simulink model "sf_ladder_logic_scheduler"  (Simulink 7.6)
settings: Solver=FixedStepDiscrete  StartTime=0.0  StopTime=10  RelTol=1e-3
model workspace (MAT data in the model file):
  deltat : Simulink.Parameter (value not decoded)
settings Model: Creator=The MathWorks Inc.
settings SolverCC: InsertRTBMode=Auto
settings OptimizationCC: InitFltsAndDblsToZero=on
settings DebuggingCC: SaveWithParameterizedLinksMsg=none  SignalResolutionControl=TryResolveAllWithWarning  InheritedTsInSrcMsg=none  MultiTaskDSMMsg=warning  MultiTaskCondExecSysMsg=none  StrictBusMsg=None
settings SFSimCC: SFSimEcho=off  SimParseCustomCode=off
settings RTWCC: IncludeERTFirstTime=on
settings GRTTargetCC: TargetFcnLib=ansi_tfl_tmw.mat

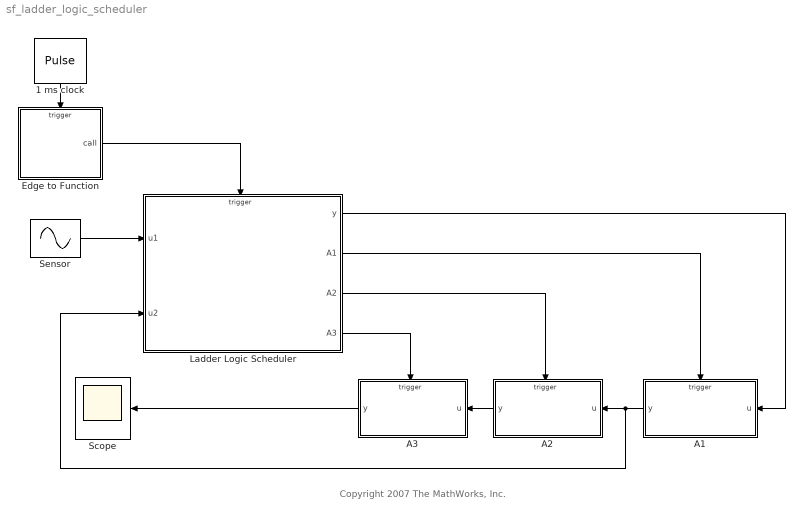
== system sf_ladder_logic_scheduler ==
  note: Copyright 2007 The MathWorks, Inc.
  1 ms clock : DiscretePulseGenerator  PulseType=Time based  Period=0.001  PulseWidth=10
  A1 : Subsystem  TreatAsAtomicUnit=on
  A2 : Subsystem  TreatAsAtomicUnit=on
  A3 : Subsystem  TreatAsAtomicUnit=on
  "Edge to Function " : Stateflow chart  TreatAsAtomicUnit=on
  Ladder Logic Scheduler : Stateflow chart  TreatAsAtomicUnit=on
  Scope : Scope
      settings: TimeRange=0.5  YMin=0  YMax=2
  Sensor : Sin  Frequency=40  Phase=-pi/8
  wires:
  Ladder Logic Scheduler/1(y) -> A1/1(u)
  Ladder Logic Scheduler/2(A1) -> A1/Trigger
  Ladder Logic Scheduler/3(A2) -> A2/Trigger
  Ladder Logic Scheduler/4(A3) -> A3/Trigger
  A1/1(y) -> Ladder Logic Scheduler/2(u2), A2/1(u)
  A2/1(y) -> A3/1(u)
  Sensor/1 -> Ladder Logic Scheduler/1(u1)
  1 ms clock/1 -> "Edge to Function "/Trigger
  "Edge to Function "/1(call) -> Ladder Logic Scheduler/Trigger
  A3/1(y) -> Scope/1

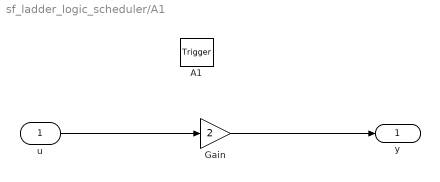
== system sf_ladder_logic_scheduler/A1 ==
  u : Inport
  A1 : TriggerPort  TriggerType=function-call
  Gain : Gain  Gain=2
  y : Outport
  wires:
  u/1 -> Gain/1
  Gain/1 -> y/1

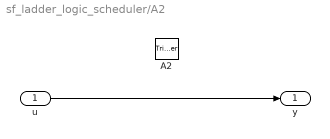
== system sf_ladder_logic_scheduler/A2 ==
  u : Inport
  A2 : TriggerPort  TriggerType=function-call
  y : Outport  InitialOutput=0
  wires:
  u/1 -> y/1

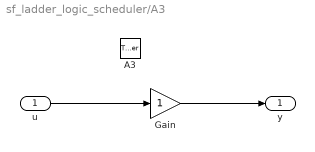
== system sf_ladder_logic_scheduler/A3 ==
  u : Inport
  A3 : TriggerPort  TriggerType=function-call
  Gain : Gain
  y : Outport
  wires:
  u/1 -> Gain/1
  Gain/1 -> y/1

== stateflow chart Ladder Logic Scheduler ==
  note: Sequencing
      | Ladder Logic
  (default) -> (junction 4) : {y=u1}
  (junction 4) -> (junction 5) [order 1] : [u1>0]
  (junction 4) -> (junction 6) [order 2]
  (junction 5) -> (junction 6) : {send(A1)}
  (junction 9) -> (junction 10) : {send(A3)}
  (junction 8) -> (junction 9) [order 1] : [(u1>0) && (u2>0)]
  (junction 7) -> (junction 8) : {send(A2)}
  (junction 8) -> (junction 10) [order 2]
  (junction 6) -> (junction 7) [order 1] : [u2 >= 0]
  (junction 6) -> (junction 8) [order 2]
  data: y output double; u1 input double; u2 input double
  events: A1 output FUNCTION_CALL_EVENT; A2 output FUNCTION_CALL_EVENT; A3 output FUNCTION_CALL_EVENT; call input FUNCTION_CALL_EVENT

== stateflow chart Edge to Function  ==
  (default) -> (junction 30) : {call;}
  events: edge input RISING_EDGE_EVENT; call output FUNCTION_CALL_EVENT
